simulink model "Assignment2"  (R2019a)
settings: Solver=FixedStepAuto  StartTime=0.0  StopTime=6  FixedStep=1  RelTol=1e-3
libraries: simulink x1
settings Model: Creator=Acer  LastModifiedBy=Acer

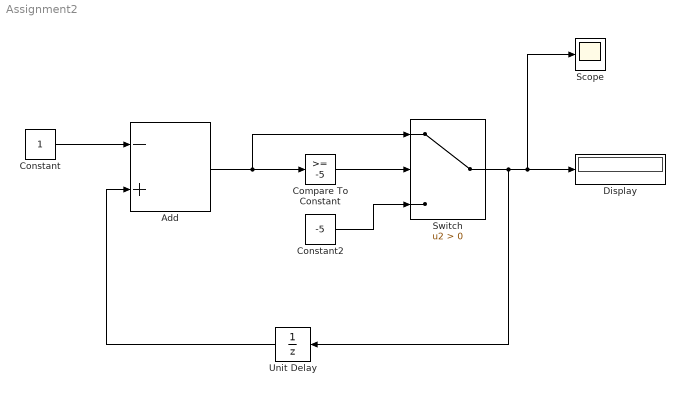
== system Assignment2 ==
  Add : Sum  Inputs=-+
  Compare To Constant : simulink/Logic and Bit Operations/Compare To Constant  relop=>=  const=-5  OutDataTypeStr=boolean
  Constant : Constant
  Constant2 : Constant  Value=-5
  Display : Display
  Scope : Scope
  Switch : Switch  Criteria=u2 > Threshold
  Unit Delay : UnitDelay  InitialCondition=1  SampleTime=-1  HasFrameUpgradeWarning=on
  wires:
  Compare To Constant/1 -> Switch/2
  Add/1 -> Switch/1, Compare To Constant/1
  Constant/1 -> Add/1
  Constant2/1 -> Switch/3
  Switch/1 -> Unit Delay/1, Scope/1, Display/1
  Unit Delay/1 -> Add/2
